simulink model "lab9_sl"  (R2021a)
settings: Solver=ode45  StartTime=0.0  StopTime=150.0  MaxStep=0.05  RelTol=1e-3
settings Model: Creator=kp46556  LastModifiedBy=kp46556

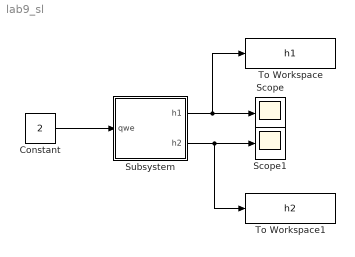
== system lab9_sl ==
  Constant : Constant  Value=2
  Scope : Scope
  Scope1 : Scope
  Subsystem : Subsystem  mask{h1=4, h2=2, S1=1, S2=2, Swy1=0.2, Swy2=0.2, g=9.81, qwe=2, f1=1, f2=1}
  To Workspace : ToWorkspace  VariableName=h1  SampleTime=-1
  To Workspace1 : ToWorkspace  VariableName=h2  SampleTime=-1
  wires:
  Constant/1 -> Subsystem/1(qwe)
  Subsystem/1(h1) -> To Workspace/1, Scope/1
  Subsystem/2(h2) -> To Workspace1/1, Scope1/1

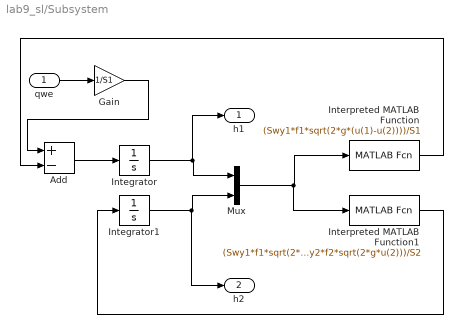
== system lab9_sl/Subsystem ==
  qwe : Inport
  Add : Sum  Inputs=+-
  Gain : Gain  Gain=1/S1
  Integrator : Integrator  InitialCondition=h1
  Integrator1 : Integrator  InitialCondition=h2
  Interpreted MATLAB Function : MATLABFcn  MATLABFcn=(Swy1*f1*sqrt(2*g*(u(1)-u(2))))/S1  OutputDimensions=1
  Interpreted MATLAB Function1 : MATLABFcn  MATLABFcn=(Swy1*f1*sqrt(2*g*(u(1)-u(2))))/S2-(Swy2*f2*sqrt(2*g*u(2)))/S2  OutputDimensions=1
  Mux : Mux  Inputs=2
  h1 : Outport
  h2 : Outport  Port=2
  wires:
  Mux/1 -> Interpreted MATLAB Function1/1, Interpreted MATLAB Function/1
  qwe/1 -> Gain/1
  Integrator/1 -> h1/1, Mux/1
  Add/1 -> Integrator/1
  Integrator1/1 -> h2/1, Mux/2
  Interpreted MATLAB Function1/1 -> Integrator1/1
  Gain/1 -> Add/1
  Interpreted MATLAB Function/1 -> Add/2
